simulink model "clack_park_transform"  (Simulink 10.2)
settings: Solver=ode45  StartTime=0.0  StopTime=0.2  RelTol=1e-3  EnableMultiTasking=on
undefined symbols (not defined in the file): DiscIntNeverNeededParam
settings Model: Creator=15070  LastModifiedBy=15070
settings DataIOCC: LimitDataPoints=on
settings OptimizationCC: ExpressionDepthLimit=2147483647
settings DebuggingCC: SolverPrmCheckMsg=warning  StateNameClashWarn=warning

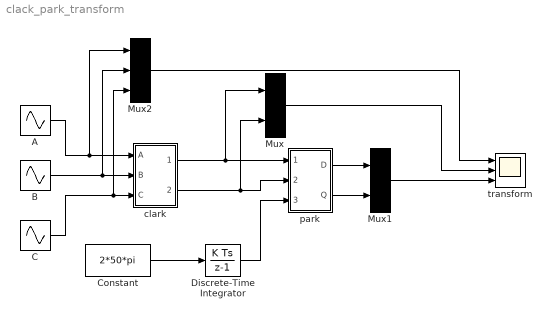
== system clack_park_transform ==
  A : Sin  Amplitude=220  Frequency=50*2*pi  SampleTime=10e-6
  B : Sin  Amplitude=220  Frequency=50*2*pi  Phase=-2/3*pi  SampleTime=10e-6
  C : Sin  Amplitude=220  Frequency=50*2*pi  Phase=2/3*pi  SampleTime=10e-6
  Constant : Constant  Value=2*50*pi
  Discrete-Time Integrator : DiscreteIntegrator  SampleTime=10e-6  ICPrevOutput=DiscIntNeverNeededParam  ICPrevScaledInput=DiscIntNeverNeededParam
  Mux : Mux  Inputs=2
  Mux1 : Mux  Inputs=2
  Mux2 : Mux  Inputs=3
  clark : Subsystem
  park : Subsystem
  transform : Scope  NumInputPorts=3
  wires:
  C/1 -> Mux2/3, clark/3(C)
  B/1 -> Mux2/2, clark/2(B)
  A/1 -> Mux2/1, clark/1(A)
  Mux/1 -> transform/2
  clark/1(Alpha) -> park/1(Alpha), Mux/1
  clark/2(Beta) -> Mux/2, park/2(Beta)
  Mux1/1 -> transform/3
  park/1(D) -> Mux1/1
  park/2(Q) -> Mux1/2
  Constant/1 -> Discrete-Time Integrator/1
  Discrete-Time Integrator/1 -> park/3(Theta)
  Mux2/1 -> transform/1

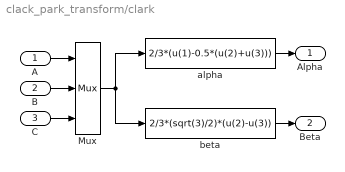
== system clack_park_transform/clark ==
  A : Inport
  B : Inport  Port=2
  C : Inport  Port=3
  Mux : Mux  Inputs=3
  alpha : Fcn  Expr=2/3*(u(1)-0.5*(u(2)+u(3)))
  beta : Fcn  Expr=2/3*(sqrt(3)/2)*(u(2)-u(3))
  Alpha : Outport
  Beta : Outport  Port=2
  wires:
  Mux/1 -> alpha/1, beta/1
  alpha/1 -> Alpha/1
  A/1 -> Mux/1
  B/1 -> Mux/2
  C/1 -> Mux/3
  beta/1 -> Beta/1

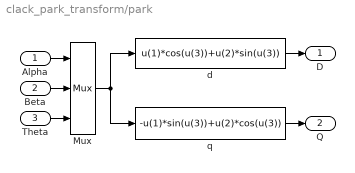
== system clack_park_transform/park ==
  Alpha : Inport
  Beta : Inport  Port=2
  Theta : Inport  Port=3
  Mux : Mux  Inputs=3
  d : Fcn  Expr=u(1)*cos(u(3))+u(2)*sin(u(3))
  q : Fcn  Expr=-u(1)*sin(u(3))+u(2)*cos(u(3))
  D : Outport
  Q : Outport  Port=2
  wires:
  Mux/1 -> d/1, q/1
  d/1 -> D/1
  Alpha/1 -> Mux/1
  Beta/1 -> Mux/2
  Theta/1 -> Mux/3
  q/1 -> Q/1
